simulink model "solar_system"  (R2024b)
settings: Solver=VariableStepAuto  StartTime=0.0  StopTime=Tsim  RelTol=1e-3
values from neighbouring files (symbols this model uses):
  G = 6.6743e-11    [main.m]
  m = [      1.98841e30 ... (first row only)    [main.m]
  Rvec0 = reshape(r0.', [], 1)    [main.m]
  Vvec0 = reshape(v0.', [], 1)    [main.m]
settings Model: Creator=amali  LastModifiedBy=amali

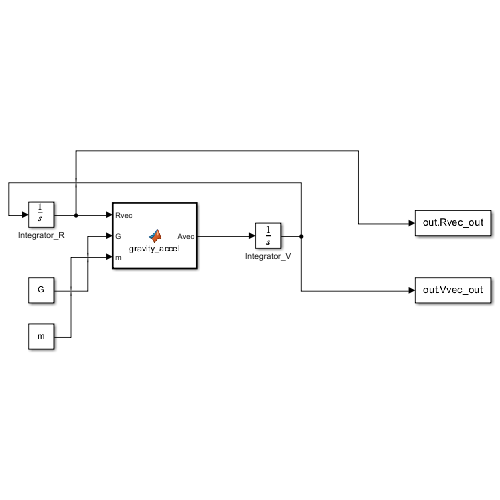
[thumbnail: Simulink's stored preview of the top-level diagram]
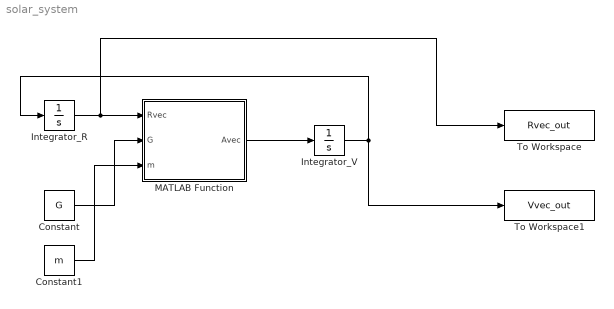
== system solar_system ==
  Constant : Constant  Value=G
  Constant1 : Constant  Value=m
  Integrator_R : Integrator  InitialCondition=Rvec0
  Integrator_V : Integrator  InitialCondition=Vvec0
  MATLAB Function : MATLAB Function  TreatAsAtomicUnit=on
  To Workspace : ToWorkspace  VariableName=Rvec_out  SaveFormat=Timeseries  SampleTime=-1
  To Workspace1 : ToWorkspace  VariableName=Vvec_out  SaveFormat=Timeseries  SampleTime=-1
  wires:
  Integrator_R/1 -> To Workspace/1, MATLAB Function/1(Rvec)
  MATLAB Function/1(Avec) -> Integrator_V/1
  Integrator_V/1 -> To Workspace1/1, Integrator_R/1
  Constant/1 -> MATLAB Function/2(G)
  Constant1/1 -> MATLAB Function/3(m)

== matlab function solar_system/MATLAB Function ==
  data: Rvec input; Avec output; G input; m input
function Avec = gravity_accel(Rvec, G, m)
%#codegen
% Calculeaza acceleratiile gravitationale (N-body)

% foloseste G si m din base workspace (init_solar.m)
N = 9;
R = reshape(Rvec, 3, N).';   % 9x3

A = zeros(N,3);

for i = 1:N
    ai = [0,0,0];
    ri = R(i,:);
    for j = 1:N
        if j == i
            continue;
        end
        d = R(j,:) - ri;
        dist = sqrt(d(1)^2 + d(2)^2 + d(3)^2);
        dist3 = dist^3 + 1e-9;   % stabilitate numerica
        ai = ai + (G*m(j)) * (d / dist3);
    end
    A(i,:) = ai;
end

Avec = reshape(A.', [], 1);   % 27x1
